simulink model "testmodel1_1102"  (R2015b)
settings: Solver=FixedStepDiscrete  StartTime=0.0  StopTime=50  FixedStep=Ts  RelTol=1e-3
PreLoadFcn:
  | Ts_IO601 = 0.001;
InitFcn:
  | Ts_IO601 = 0.001;
  | Ts=0.001;
libraries: canmsglib x11, speedgoatlib_IO601 x10, slrtlib x7, simulink x2
settings Model: Creator=lab2  LastModifiedBy=1SMARTe
settings SolverCC: EnableConcurrentExecution=on
settings DataIOCC: SaveFormat=Array
settings OptimizationCC: BlockReduction=off  OptimizeBlockIOStorage=off  BufferReuse=off  GlobalBufferReuse=off  ExpressionFolding=off  LocalBlockOutputs=off
settings DebuggingCC: UnconnectedInputMsg=none  UnconnectedOutputMsg=none  UnconnectedLineMsg=none
settings HardwareCC: ProdBitPerPointer=32  ProdLargestAtomicFloat=None  ProdWordSize=32  ProdLongLongMode=on  ProdHWDeviceType=Generic->32-bit x86 compatible
settings RTWCC: SystemTargetFile=slrt.tlc  TemplateMakefile=slrt_default_tmf  Description=Simulink Real-Time  RTWCompilerOptimization=on
settings ConfigComp: CovModelRefEnable=Off

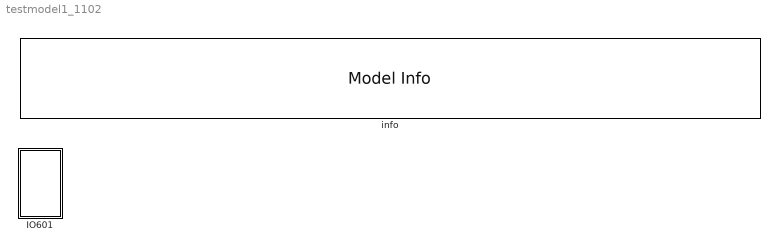
== system testmodel1_1102 ==
  IO601 : Subsystem
  info : simulink/Model-Wide Utilities/Model Info  Frame=on  DisplayStringWithTags=|  HorizontalTextAlignment=Left  LeftAlignmentValue=0.02  SourceBlockDiagram=testmodel1_1102  TagMaxNumber=20
      | SPEEDGOAT Simulink Real-Time  test model for Real-time target machine (SN2820)
      | prepared by Speedgoat with MATLAB R2015a
      | 
      | Build date: %<Created>

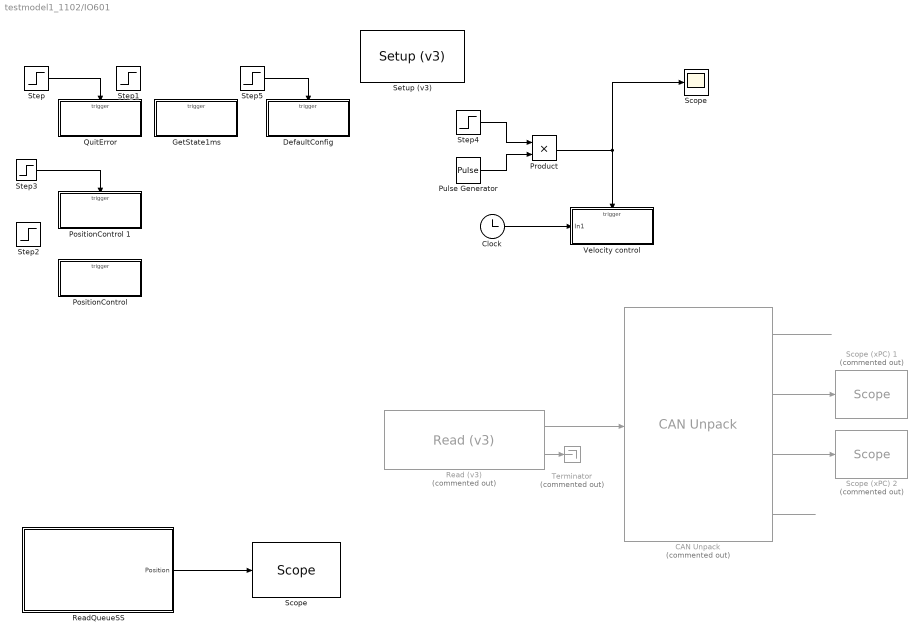
== system testmodel1_1102/IO601 ==
  CAN Unpack : canmsglib/CAN Unpack  Commented=on  MsgList=(none)  MsgName=Test message  MsgIDType=Standard (11-bit identifier)  MsgIdentifier=hex2dec('703')  MsgLength=6  SignalInfo=Dlen$0$8$1$2$1$0$1$0$-Inf$Inf$#Cmd$8$8$1$2$1$0$1$0$-Inf$Inf$#Position$16$32$1$1$1$0$1$0$-Inf$Inf$#  NSignals=3  IDPort=on  TimestampPort=off  ErrorPort=off  RemotePort=off  LengthPort=off  StatusPort=off  StartBits=str2num('[int32(0);int32(8);int32(16)]')  SignalSizes=str2num('[int32(8);int32(8);int32(32)]')  ByteOrders=str2num('[int32(1);int32(1);int32(1)]')  DataTypes=str2num('[int32(2);int32(2);int32(1)]')  MultiplexTypes=str2num('[int32(1);int32(1);int32(1)]')  MultiplexValues=str2num('[double(0);double(0);double(0)]')  Factors=str2num('[double(1);double(1);double(1)]')  Offsets=str2num('[double(0);double(0);double(0)]')  Minimums=str2num('[double(-Inf);double(-Inf);double(-Inf)]')  Maximums=str2num('[double(Inf);double(Inf);double(Inf)]')
  Clock : Clock
  DefaultConfig : Subsystem  TreatAsAtomicUnit=on
  GetState1ms : Subsystem  TreatAsAtomicUnit=on
  "PositionControl " : Subsystem  TreatAsAtomicUnit=on
  PositionControl 1 : Subsystem  TreatAsAtomicUnit=on
  Product : Product
  Pulse Generator : DiscretePulseGenerator  PulseType=Time based  Period=Ts*10  PulseWidth=10  PhaseDelay=10  SampleTime=Ts_IO601
  QuitError : Subsystem  TreatAsAtomicUnit=on
  Read (v3) : speedgoatlib_IO601/Read (v3)  Commented=on  id=1  outputFormat=Vector of CAN_MESSAGE  port1=on  port2=off  depth1=1  depth2=1  sampletime=-1  pciSlot=-1
  ReadQueueSS : Subsystem
  Scope : Scope
  "Scope " : slrtlib/Displays and Logging/Scope   scopeno=4  scopetype=Target  autostart=on  viewmode=Graphical sliding  formatstr='%15.6f'  grid=on  ylimits=[-90000,90000]  nosamples=10/Ts  noprepostsamples=0  interleave=1  triggermode=FreeRun  triggersignal=1  trigsignalfromport=off  triggerlevel=0.0  triggerslope=Either  triggerscope=1  triggersample=0  filename=data.dat  mode=Lazy  writesize=512  autorestart=off  dynamicfilemode=off  maxwritefilesize=512*1024^2
  Scope (xPC) 1 : slrtlib/Displays and Logging/Scope   Commented=on  scopeno=1  scopetype=Target  autostart=on  viewmode=Numerical  formatstr='%15.6f'  grid=on  ylimits=[0,0]  nosamples=1000  noprepostsamples=0  interleave=2  triggermode=FreeRun  triggersignal=1  trigsignalfromport=off  triggerlevel=0.0  triggerslope=Rising  triggerscope=1  triggersample=0  filename=data.dat  mode=Lazy  writesize=512  autorestart=off  dynamicfilemode=off  maxwritefilesize=512*1024^2
  Scope (xPC) 2 : slrtlib/Displays and Logging/Scope   Commented=on  scopeno=3  scopetype=Target  autostart=on  viewmode=Graphical rolling  formatstr='%15.6f'  grid=on  ylimits=[0,0]  nosamples=1000  noprepostsamples=0  interleave=2  triggermode=FreeRun  triggersignal=1  trigsignalfromport=off  triggerlevel=0.0  triggerslope=Rising  triggerscope=1  triggersample=0  filename=data.dat  mode=Lazy  writesize=512  autorestart=off  dynamicfilemode=off  maxwritefilesize=512*1024^2
  Setup (v3) : speedgoatlib_IO601/Setup (v3)  id=1  can1enable=on  can1bus=Highspeed  can1Baudrate=1 MBaud  can1UserBR=[1,1,5,2]  stdAcc1=[0,0,0,0]  extAcc1=[0,0,0,0]  can2enable=on  can2bus=Highspeed  can2Baudrate=1 MBaud  can2UserBR=[1,1,5,2]  stdAcc2=[0,0,0,0]  extAcc2=[0,0,0,0]  pciSlot=-1
  Step : Step  SampleTime=Ts
  Step1 : Step  Time=2  Before=1  After=0  SampleTime=Ts
  Step2 : Step  Time=8  SampleTime=Ts
  Step3 : Step  Time=5  SampleTime=Ts
  Step4 : Step  Time=30  Before=1  After=0  SampleTime=0
  Step5 : Step  Time=40  SampleTime=Ts
  Terminator : Terminator  Commented=on
  Velocity control : Subsystem  TreatAsAtomicUnit=on
  wires:
  CAN Unpack/1 -> ?
  CAN Unpack/2 -> Scope (xPC) 1/1
  CAN Unpack/3 -> Scope (xPC) 2/1
  CAN Unpack/4 -> ?
  Step/1 -> QuitError/Trigger
  Clock/1 -> Velocity control/1(In1)
  Read (v3)/1 -> CAN Unpack/1
  Read (v3)/2 -> Terminator/1
  Step4/1 -> Product/1
  Pulse Generator/1 -> Product/2
  Step3/1 -> PositionControl 1/Trigger
  Step5/1 -> DefaultConfig/Trigger
  Product/1 -> Velocity control/Trigger, Scope/1
  ReadQueueSS/1(Position) -> "Scope "/1

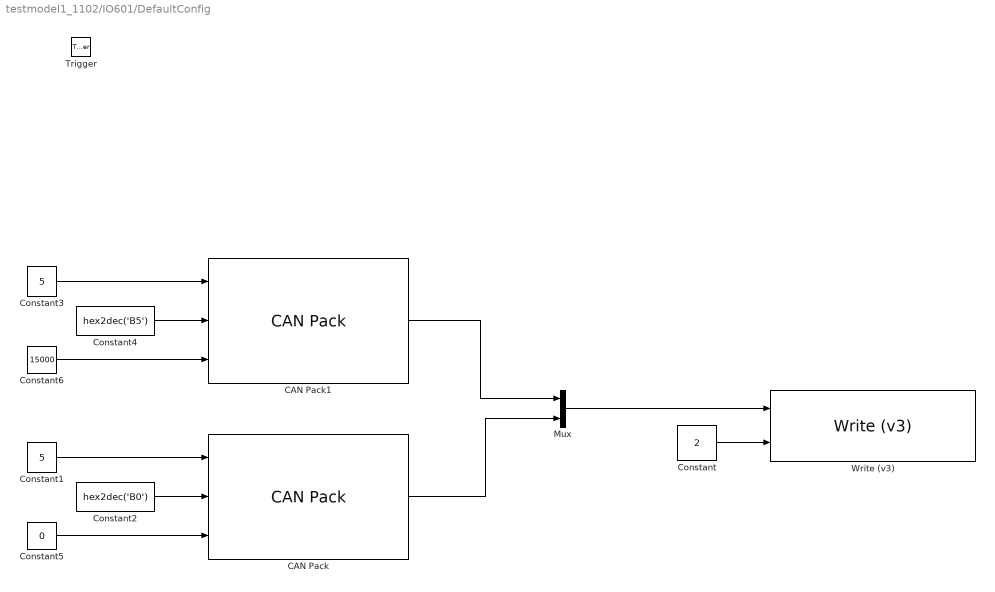
== system testmodel1_1102/IO601/DefaultConfig ==
  Trigger : TriggerPort
  CAN Pack : canmsglib/CAN Pack  MsgList=(none)  MsgName=Position Msg  MsgIDType=Standard (11-bit identifier)  MsgIdentifier=hex2dec('503')  MsgLength=6  SignalInfo=Signal1$0$8$1$2$1$0$1$0$-Inf$Inf$#Signal2$8$8$1$2$1$0$1$0$-Inf$Inf$#Signal3$16$32$1$1$1$0$1$0$-Inf$Inf$#  NSignals=3  StartBits=str2num('[int32(0);int32(8);int32(16)]')  SignalSizes=str2num('[int32(8);int32(8);int32(32)]')  ByteOrders=str2num('[int32(1);int32(1);int32(1)]')  DataTypes=str2num('[int32(2);int32(2);int32(1)]')  MultiplexTypes=str2num('[int32(1);int32(1);int32(1)]')  MultiplexValues=str2num('[double(0);double(0);double(0)]')  Factors=str2num('[double(1);double(1);double(1)]')  Offsets=str2num('[double(0);double(0);double(0)]')  Minimums=str2num('[double(-Inf);double(-Inf);double(-Inf)]')  Maximums=str2num('[double(Inf);double(Inf);double(Inf)]')  Remote=off
      settings: DataFormat=manually specified signals
  CAN Pack1 : canmsglib/CAN Pack  MsgList=(none)  MsgName=Position Msg  MsgIDType=Standard (11-bit identifier)  MsgIdentifier=hex2dec('503')  MsgLength=6  SignalInfo=Signal1$0$8$1$2$1$0$1$0$-Inf$Inf$#Signal2$8$8$1$2$1$0$1$0$-Inf$Inf$#Signal3$16$32$1$1$1$0$1$0$-Inf$Inf$#  NSignals=3  StartBits=str2num('[int32(0);int32(8);int32(16)]')  SignalSizes=str2num('[int32(8);int32(8);int32(32)]')  ByteOrders=str2num('[int32(1);int32(1);int32(1)]')  DataTypes=str2num('[int32(2);int32(2);int32(1)]')  MultiplexTypes=str2num('[int32(1);int32(1);int32(1)]')  MultiplexValues=str2num('[double(0);double(0);double(0)]')  Factors=str2num('[double(1);double(1);double(1)]')  Offsets=str2num('[double(0);double(0);double(0)]')  Minimums=str2num('[double(-Inf);double(-Inf);double(-Inf)]')  Maximums=str2num('[double(Inf);double(Inf);double(Inf)]')  Remote=off
      settings: DataFormat=manually specified signals
  Constant : Constant  Value=2
  Constant1 : Constant  Value=5
  Constant2 : Constant  Value=hex2dec('B0')
  Constant3 : Constant  Value=5
  Constant4 : Constant  Value=hex2dec('B5')
  Constant5 : Constant  Value=0
  Constant6 : Constant  Value=15000
  Mux : Mux  Inputs=2
  Write (v3) : speedgoatlib_IO601/Write (v3)  Priority=1  id=1  sampletime=-1  pciSlot=-1  inputType=CAN_MESSAGE plus count  port=1  maxMsg=2  status=off  init=[]  term=[]
  wires:
  CAN Pack/1 -> Mux/2
  Constant/1 -> Write (v3)/2
  Constant1/1 -> CAN Pack/1
  Constant2/1 -> CAN Pack/2
  Constant5/1 -> CAN Pack/3
  CAN Pack1/1 -> Mux/1
  Constant3/1 -> CAN Pack1/1
  Constant4/1 -> CAN Pack1/2
  Constant6/1 -> CAN Pack1/3
  Mux/1 -> Write (v3)/1

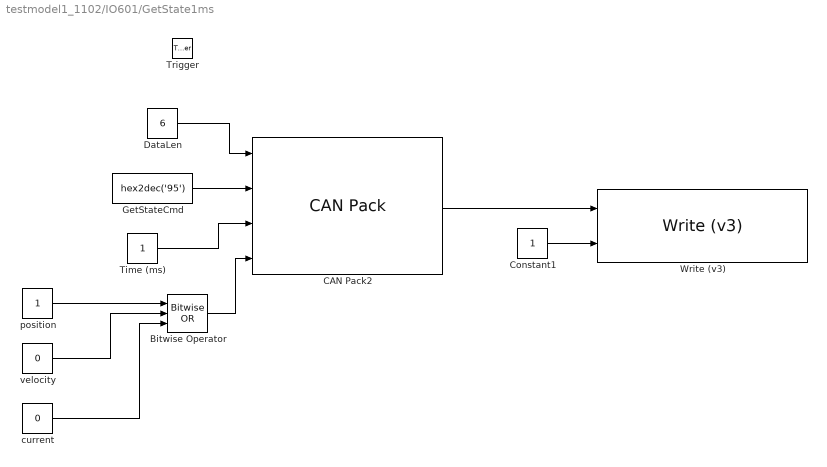
== system testmodel1_1102/IO601/GetState1ms ==
  Trigger : TriggerPort  TriggerType=falling
  Bitwise Operator : simulink/Logic and Bit Operations/Bitwise Operator  logicop=OR  UseBitMask=off  NumInputPorts=3  BitMask=bin2dec('11011001')  BitMaskRealWorld=Stored Integer
  CAN Pack2 : canmsglib/CAN Pack  MsgList=(none)  MsgName=GetState  MsgIDType=Standard (11-bit identifier)  MsgIdentifier=hex2dec('503')  MsgLength=7  SignalInfo=Signal1$0$8$1$2$1$0$1$0$-Inf$Inf$#Signal2$8$8$1$2$1$0$1$0$-Inf$Inf$#time$16$32$1$2$1$0$1$0$-Inf$Inf$#mode$48$8$1$2$1$0$1$0$-Inf$Inf$#  NSignals=4  StartBits=str2num('[int32(0);int32(8);int32(16);int32(48)]')  SignalSizes=str2num('[int32(8);int32(8);int32(32);int32(8)]')  ByteOrders=str2num('[int32(1);int32(1);int32(1);int32(1)]')  DataTypes=str2num('[int32(2);int32(2);int32(2);int32(2)]')  MultiplexTypes=str2num('[int32(1);int32(1);int32(1);int32(1)]')  MultiplexValues=str2num('[double(0);double(0);double(0);double(0)]')  Factors=str2num('[double(1);double(1);double(1);double(1)]')  Offsets=str2num('[double(0);double(0);double(0);double(0)]')  Minimums=str2num('[double(-Inf);double(-Inf);double(-Inf);double(-Inf)]')  Maximums=str2num('[double(Inf);double(Inf);double(Inf);double(Inf)]')  Remote=off
      settings: DataFormat=manually specified signals
  Constant1 : Constant
  DataLen : Constant  Value=6
  GetStateCmd : Constant  Value=hex2dec('95')
  Time (ms) : Constant
  Write (v3) : speedgoatlib_IO601/Write (v3)  Priority=1  id=1  sampletime=-1  pciSlot=-1  inputType=CAN_MESSAGE plus count  port=1  maxMsg=1  status=off  init=[]  term=[]
  current : Constant  Value=0  OutDataTypeStr=uint8
  position : Constant  OutDataTypeStr=uint8
  velocity : Constant  Value=0  OutDataTypeStr=uint8
  wires:
  Constant1/1 -> Write (v3)/2
  Time (ms)/1 -> CAN Pack2/3
  DataLen/1 -> CAN Pack2/1
  GetStateCmd/1 -> CAN Pack2/2
  CAN Pack2/1 -> Write (v3)/1
  position/1 -> Bitwise Operator/1
  Bitwise Operator/1 -> CAN Pack2/4
  velocity/1 -> Bitwise Operator/2
  current/1 -> Bitwise Operator/3

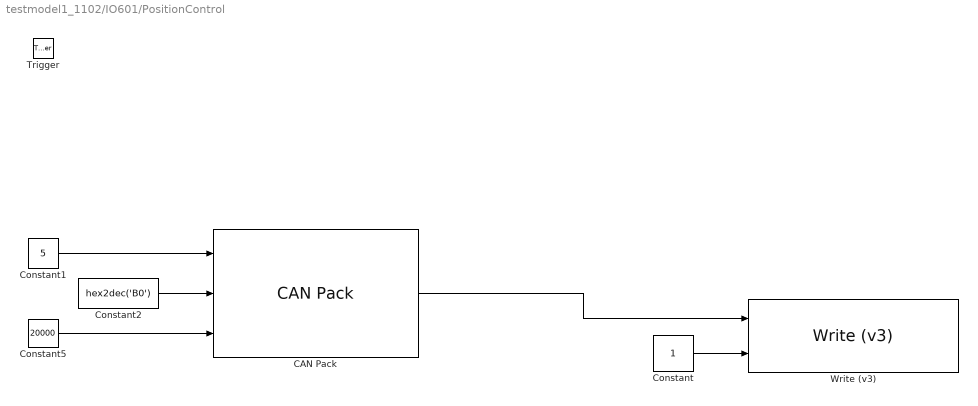
== system testmodel1_1102/IO601/PositionControl  ==
  Trigger : TriggerPort
  CAN Pack : canmsglib/CAN Pack  MsgList=(none)  MsgName=Position Msg  MsgIDType=Standard (11-bit identifier)  MsgIdentifier=hex2dec('503')  MsgLength=6  SignalInfo=Signal1$0$8$1$2$1$0$1$0$-Inf$Inf$#Signal2$8$8$1$2$1$0$1$0$-Inf$Inf$#Signal3$16$32$1$1$1$0$1$0$-Inf$Inf$#  NSignals=3  StartBits=str2num('[int32(0);int32(8);int32(16)]')  SignalSizes=str2num('[int32(8);int32(8);int32(32)]')  ByteOrders=str2num('[int32(1);int32(1);int32(1)]')  DataTypes=str2num('[int32(2);int32(2);int32(1)]')  MultiplexTypes=str2num('[int32(1);int32(1);int32(1)]')  MultiplexValues=str2num('[double(0);double(0);double(0)]')  Factors=str2num('[double(1);double(1);double(1)]')  Offsets=str2num('[double(0);double(0);double(0)]')  Minimums=str2num('[double(-Inf);double(-Inf);double(-Inf)]')  Maximums=str2num('[double(Inf);double(Inf);double(Inf)]')  Remote=off
      settings: DataFormat=manually specified signals
  Constant : Constant
  Constant1 : Constant  Value=5
  Constant2 : Constant  Value=hex2dec('B0')
  Constant5 : Constant  Value=20000
  Write (v3) : speedgoatlib_IO601/Write (v3)  Priority=1  id=1  sampletime=-1  pciSlot=-1  inputType=CAN_MESSAGE plus count  port=1  maxMsg=1  status=off  init=[]  term=[]
  wires:
  CAN Pack/1 -> Write (v3)/1
  Constant/1 -> Write (v3)/2
  Constant1/1 -> CAN Pack/1
  Constant2/1 -> CAN Pack/2
  Constant5/1 -> CAN Pack/3

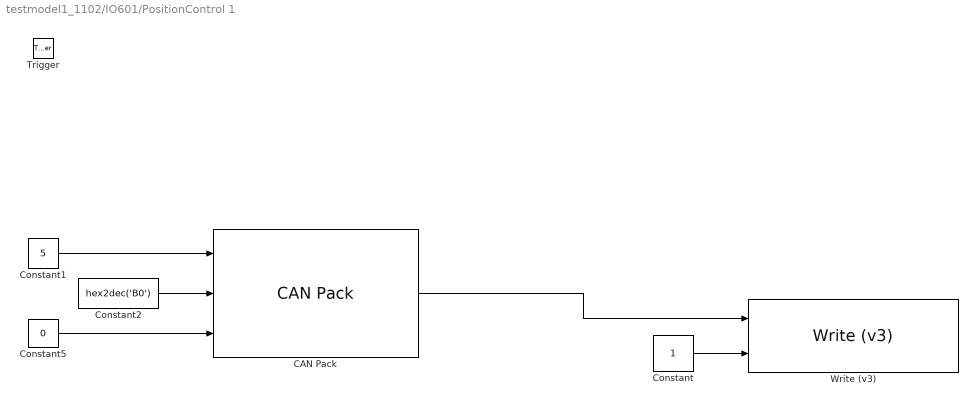
== system testmodel1_1102/IO601/PositionControl 1 ==
  Trigger : TriggerPort
  CAN Pack : canmsglib/CAN Pack  MsgList=(none)  MsgName=Position Msg  MsgIDType=Standard (11-bit identifier)  MsgIdentifier=1283  MsgLength=6  SignalInfo=Signal1$0$8$1$2$1$0$1$0$-Inf$Inf$#Signal2$8$8$1$2$1$0$1$0$-Inf$Inf$#Signal3$16$32$1$1$1$0$1$0$-Inf$Inf$#  NSignals=3  StartBits=str2num('[int32(0);int32(8);int32(16)]')  SignalSizes=str2num('[int32(8);int32(8);int32(32)]')  ByteOrders=str2num('[int32(1);int32(1);int32(1)]')  DataTypes=str2num('[int32(2);int32(2);int32(1)]')  MultiplexTypes=str2num('[int32(1);int32(1);int32(1)]')  MultiplexValues=str2num('[double(0);double(0);double(0)]')  Factors=str2num('[double(1);double(1);double(1)]')  Offsets=str2num('[double(0);double(0);double(0)]')  Minimums=str2num('[double(-Inf);double(-Inf);double(-Inf)]')  Maximums=str2num('[double(Inf);double(Inf);double(Inf)]')  Remote=off
      settings: DataFormat=manually specified signals
  Constant : Constant
  Constant1 : Constant  Value=5
  Constant2 : Constant  Value=hex2dec('B0')
  Constant5 : Constant  Value=0
  Write (v3) : speedgoatlib_IO601/Write (v3)  Priority=1  id=1  sampletime=-1  pciSlot=-1  inputType=CAN_MESSAGE plus count  port=1  maxMsg=1  status=off  init=[]  term=[]
  wires:
  CAN Pack/1 -> Write (v3)/1
  Constant/1 -> Write (v3)/2
  Constant1/1 -> CAN Pack/1
  Constant2/1 -> CAN Pack/2
  Constant5/1 -> CAN Pack/3

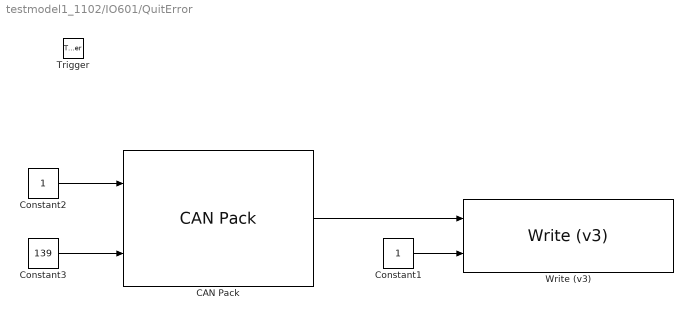
== system testmodel1_1102/IO601/QuitError ==
  Trigger : TriggerPort
  CAN Pack : canmsglib/CAN Pack  MsgList=(none)  MsgName=QuitError  MsgIDType=Standard (11-bit identifier)  MsgIdentifier=hex2dec('503')  MsgLength=2  SignalInfo=Signal1$0$8$1$2$1$0$1$0$-Inf$Inf$#Signal2$8$8$1$2$1$0$1$0$-Inf$Inf$#  NSignals=2  StartBits=str2num('[int32(0);int32(8)]')  SignalSizes=str2num('[int32(8);int32(8)]')  ByteOrders=str2num('[int32(1);int32(1)]')  DataTypes=str2num('[int32(2);int32(2)]')  MultiplexTypes=str2num('[int32(1);int32(1)]')  MultiplexValues=str2num('[double(0);double(0)]')  Factors=str2num('[double(1);double(1)]')  Offsets=str2num('[double(0);double(0)]')  Minimums=str2num('[double(-Inf);double(-Inf)]')  Maximums=str2num('[double(Inf);double(Inf)]')  Remote=off
      settings: DataFormat=manually specified signals
  Constant1 : Constant
  Constant2 : Constant
  Constant3 : Constant  Value=139
  Write (v3) : speedgoatlib_IO601/Write (v3)  Priority=1  id=1  sampletime=-1  pciSlot=-1  inputType=CAN_MESSAGE plus count  port=1  maxMsg=1  status=off  init=[]  term=[]
  wires:
  Constant3/1 -> CAN Pack/2
  Constant2/1 -> CAN Pack/1
  CAN Pack/1 -> Write (v3)/1
  Constant1/1 -> Write (v3)/2

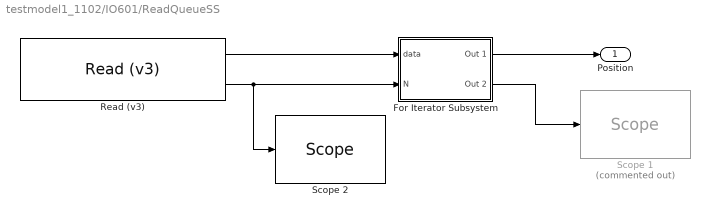
== system testmodel1_1102/IO601/ReadQueueSS ==
  For Iterator Subsystem : Subsystem  TreatAsAtomicUnit=on
  Read (v3) : speedgoatlib_IO601/Read (v3)  id=1  outputFormat=Vector of CAN_MESSAGE  port1=on  port2=off  depth1=50  depth2=4  sampletime=-1  pciSlot=-1
  Scope 1 : slrtlib/Displays and Logging/Scope   Commented=on  scopeno=2  scopetype=Target  autostart=on  viewmode=Numerical  formatstr='%15.6f'  grid=on  ylimits=[0,0]  nosamples=3  noprepostsamples=0  interleave=1  triggermode=FreeRun  triggersignal=1  trigsignalfromport=off  triggerlevel=0.0  triggerslope=Either  triggerscope=1  triggersample=0  filename=data.dat  mode=Lazy  writesize=512  autorestart=off  dynamicfilemode=off  maxwritefilesize=512*1024^2
  Scope 2 : slrtlib/Displays and Logging/Scope   scopeno=1  scopetype=Target  autostart=on  viewmode=Numerical  formatstr='%15.6f'  grid=on  ylimits=[0,0]  nosamples=1000  noprepostsamples=0  interleave=1  triggermode=FreeRun  triggersignal=1  trigsignalfromport=off  triggerlevel=0.0  triggerslope=Either  triggerscope=1  triggersample=0  filename=data.dat  mode=Lazy  writesize=512  autorestart=off  dynamicfilemode=off  maxwritefilesize=512*1024^2
  Position : Outport
  wires:
  Read (v3)/1 -> For Iterator Subsystem/1(data)
  Read (v3)/2 -> Scope 2/1, For Iterator Subsystem/2(N)
  For Iterator Subsystem/2(Out 2) -> Scope 1/1
  For Iterator Subsystem/1(Out 1) -> Position/1

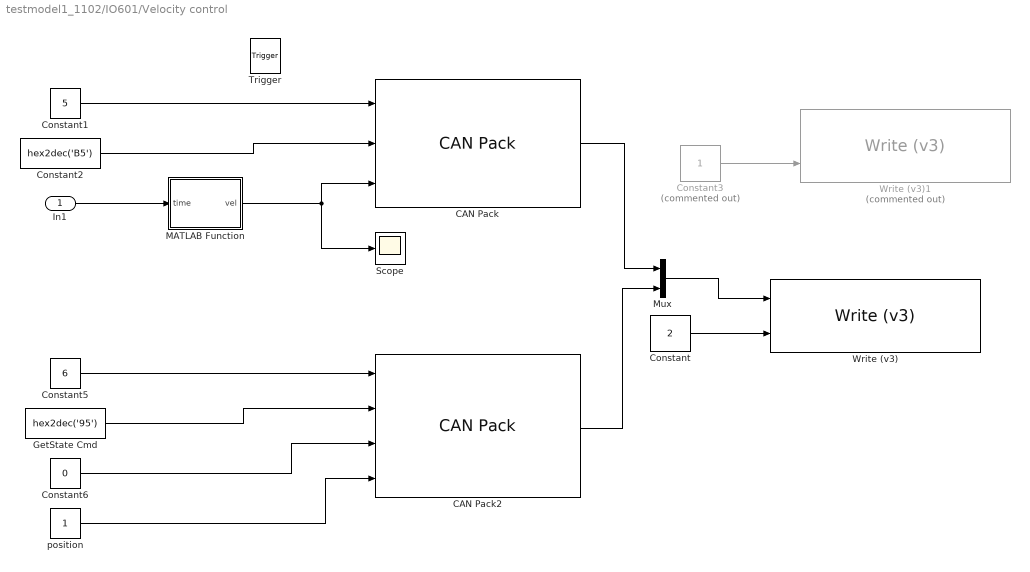
== system testmodel1_1102/IO601/Velocity control ==
  In1 : Inport
  Trigger : TriggerPort
  CAN Pack : canmsglib/CAN Pack  MsgList=(none)  MsgName=Position Msg  MsgIDType=Standard (11-bit identifier)  MsgIdentifier=hex2dec('503')  MsgLength=6  SignalInfo=Signal1$0$8$1$2$1$0$1$0$-Inf$Inf$#Signal2$8$8$1$2$1$0$1$0$-Inf$Inf$#Signal3$16$32$1$1$1$0$1$0$-Inf$Inf$#  NSignals=3  StartBits=str2num('[int32(0);int32(8);int32(16)]')  SignalSizes=str2num('[int32(8);int32(8);int32(32)]')  ByteOrders=str2num('[int32(1);int32(1);int32(1)]')  DataTypes=str2num('[int32(2);int32(2);int32(1)]')  MultiplexTypes=str2num('[int32(1);int32(1);int32(1)]')  MultiplexValues=str2num('[double(0);double(0);double(0)]')  Factors=str2num('[double(1);double(1);double(1)]')  Offsets=str2num('[double(0);double(0);double(0)]')  Minimums=str2num('[double(-Inf);double(-Inf);double(-Inf)]')  Maximums=str2num('[double(Inf);double(Inf);double(Inf)]')  Remote=off
      settings: DataFormat=manually specified signals
  CAN Pack2 : canmsglib/CAN Pack  MsgList=(none)  MsgName=GetState  MsgIDType=Standard (11-bit identifier)  MsgIdentifier=hex2dec('503')  MsgLength=7  SignalInfo=Signal1$0$8$1$2$1$0$1$0$-Inf$Inf$#Signal2$8$8$1$2$1$0$1$0$-Inf$Inf$#time$16$32$1$2$1$0$1$0$-Inf$Inf$#mode$48$8$1$2$1$0$1$0$-Inf$Inf$#  NSignals=4  StartBits=str2num('[int32(0);int32(8);int32(16);int32(48)]')  SignalSizes=str2num('[int32(8);int32(8);int32(32);int32(8)]')  ByteOrders=str2num('[int32(1);int32(1);int32(1);int32(1)]')  DataTypes=str2num('[int32(2);int32(2);int32(2);int32(2)]')  MultiplexTypes=str2num('[int32(1);int32(1);int32(1);int32(1)]')  MultiplexValues=str2num('[double(0);double(0);double(0);double(0)]')  Factors=str2num('[double(1);double(1);double(1);double(1)]')  Offsets=str2num('[double(0);double(0);double(0);double(0)]')  Minimums=str2num('[double(-Inf);double(-Inf);double(-Inf);double(-Inf)]')  Maximums=str2num('[double(Inf);double(Inf);double(Inf);double(Inf)]')  Remote=off
      settings: DataFormat=manually specified signals
  Constant : Constant  Value=2
  Constant1 : Constant  Value=5
  Constant2 : Constant  Value=hex2dec('B5')
  Constant3 : Constant  Commented=on
  Constant5 : Constant  Value=6
  Constant6 : Constant  Value=0
  GetState Cmd : Constant  Value=hex2dec('95')
  MATLAB Function : MATLAB Function  TreatAsAtomicUnit=on
  Mux : Mux  Inputs=2
  Scope : Scope
  Write (v3) : speedgoatlib_IO601/Write (v3)  Priority=1  id=1  sampletime=-1  pciSlot=-1  inputType=CAN_MESSAGE plus count  port=1  maxMsg=2  status=off  init=[]  term=[]
  Write (v3)1 : speedgoatlib_IO601/Write (v3)  Priority=1  Commented=on  id=1  sampletime=-1  pciSlot=-1  inputType=CAN_MESSAGE plus count  port=1  maxMsg=1  status=off  init=[]  term=[]
  position : Constant  OutDataTypeStr=uint8
  wires:
  Constant/1 -> Write (v3)/2
  Constant1/1 -> CAN Pack/1
  Constant2/1 -> CAN Pack/2
  In1/1 -> MATLAB Function/1(time)
  MATLAB Function/1(vel) -> CAN Pack/3, Scope/1
  Constant6/1 -> CAN Pack2/3
  Constant5/1 -> CAN Pack2/1
  GetState Cmd/1 -> CAN Pack2/2
  position/1 -> CAN Pack2/4
  CAN Pack/1 -> Mux/1
  CAN Pack2/1 -> Mux/2
  Mux/1 -> Write (v3)/1
  Constant3/1 -> Write (v3)1/2

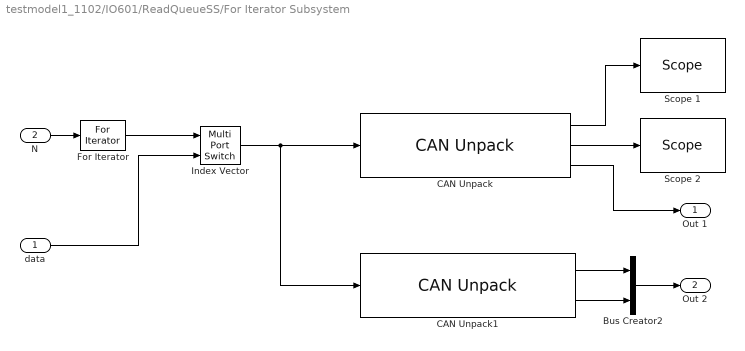
== system testmodel1_1102/IO601/ReadQueueSS/For Iterator Subsystem ==
  data : Inport
  N : Inport  Port=2
  Bus Creator2 : BusCreator  Inputs=2
  CAN Unpack : canmsglib/CAN Unpack  MsgList=(none)  MsgName=Message20  MsgIDType=Standard (11-bit identifier)  MsgIdentifier=hex2dec('703')  MsgLength=8  SignalInfo=DLen$0$8$1$2$1$0$1$0$-Inf$Inf$#Cmd$8$8$1$2$1$0$1$0$-Inf$Inf$#Position$16$32$1$1$1$0$1$0$-Inf$Inf$#  NSignals=3  IDPort=off  TimestampPort=off  ErrorPort=off  RemotePort=off  LengthPort=off  StatusPort=off  StartBits=str2num('[int32(0);int32(8);int32(16)]')  SignalSizes=str2num('[int32(8);int32(8);int32(32)]')  ByteOrders=str2num('[int32(1);int32(1);int32(1)]')  DataTypes=str2num('[int32(2);int32(2);int32(1)]')  MultiplexTypes=str2num('[int32(1);int32(1);int32(1)]')  MultiplexValues=str2num('[double(0);double(0);double(0)]')  Factors=str2num('[double(1);double(1);double(1)]')  Offsets=str2num('[double(0);double(0);double(0)]')  Minimums=str2num('[double(-Inf);double(-Inf);double(-Inf)]')  Maximums=str2num('[double(Inf);double(Inf);double(Inf)]')
  CAN Unpack1 : canmsglib/CAN Unpack  MsgList=(none)  MsgName=Message21  MsgIDType=Standard (11-bit identifier)  MsgIdentifier=33  MsgLength=4  SignalInfo=Signal3$0$16$1$1$1$0$1$0$-Inf$Inf$#Signal4$16$16$1$1$1$0$1$0$-Inf$Inf$#  NSignals=2  IDPort=off  TimestampPort=off  ErrorPort=off  RemotePort=off  LengthPort=off  StatusPort=off  StartBits=str2num('[int32(0);int32(16)]')  SignalSizes=str2num('[int32(16);int32(16)]')  ByteOrders=str2num('[int32(1);int32(1)]')  DataTypes=str2num('[int32(1);int32(1)]')  MultiplexTypes=str2num('[int32(1);int32(1)]')  MultiplexValues=str2num('[double(0);double(0)]')  Factors=str2num('[double(1);double(1)]')  Offsets=str2num('[double(0);double(0)]')  Minimums=str2num('[double(-Inf);double(-Inf)]')  Maximums=str2num('[double(Inf);double(Inf)]')
  For Iterator : ForIterator  IterationSource=external  IterationLimit=20  IterationVariableDataType=int8
  Index Vector : MultiPortSwitch  Inputs=1
  Scope 1 : slrtlib/Displays and Logging/Scope   scopeno=3  scopetype=Target  autostart=on  viewmode=Numerical  formatstr='%15.6f'  grid=on  ylimits=[0,0]  nosamples=1000  noprepostsamples=0  interleave=1  triggermode=FreeRun  triggersignal=1  trigsignalfromport=off  triggerlevel=0.0  triggerslope=Either  triggerscope=1  triggersample=0  filename=data.dat  mode=Lazy  writesize=512  autorestart=off  dynamicfilemode=off  maxwritefilesize=512*1024^2
  Scope 2 : slrtlib/Displays and Logging/Scope   scopeno=2  scopetype=Target  autostart=on  viewmode=Numerical  formatstr='%15.6f'  grid=on  ylimits=[0,0]  nosamples=1000  noprepostsamples=0  interleave=1  triggermode=FreeRun  triggersignal=1  trigsignalfromport=off  triggerlevel=0.0  triggerslope=Either  triggerscope=1  triggersample=0  filename=data.dat  mode=Lazy  writesize=512  autorestart=off  dynamicfilemode=off  maxwritefilesize=512*1024^2
  Out 1 : Outport
  Out 2 : Outport  Port=2
  wires:
  Index Vector/1 -> CAN Unpack1/1, CAN Unpack/1
  For Iterator/1 -> Index Vector/1
  data/1 -> Index Vector/2
  Bus Creator2/1 -> Out 2/1
  CAN Unpack1/1 -> Bus Creator2/1
  CAN Unpack1/2 -> Bus Creator2/2
  N/1 -> For Iterator/1
  CAN Unpack/2 -> Scope 2/1
  CAN Unpack/3 -> Out 1/1
  CAN Unpack/1 -> Scope 1/1

== matlab function testmodel1_1102/IO601/Velocity control/MATLAB Function ==
  data: time input; vel output
function vel  = fcn(time)
%#codegen
vel = 15000*sin(2*pi*time/10);
% if cp > 0
%     vel = 90000;
% else
%     vel = -90000;
% end
end
